simulink model "utpr_model_complex_22"  (R2023b)
settings: Solver=FixedStepAuto  StartTime=0  StopTime=8  FixedStep=0.01  RelTol=1e-2  AbsTol=1e-3  EnableMultiTasking=on
values from neighbouring files (symbols this model uses):
  link1_m = 1.915 * (rand_para(1,1) + 1)    [utpr_model_complex_para.m]
  link2_m = 1.469 * (rand_para(3,1) + 1)    [utpr_model_complex_para.m]
  link3_m = 1.141 * (rand_para(5,1) + 1)    [utpr_model_complex_para.m]
  N = 50    [utpr_lqr.m]    (also in utpr_mpc.m = 100)
undefined symbols (not defined in the file or in its folder): X, Y, Z
libraries: sm_lib x28, nesl_utility x24, simulink x1
settings Model: Creator=李东昊  LastModifiedBy=12720
settings SolverCC: AutoScaleAbsTol=off  AlgebraicLoopSolver=TrustRegion  MaxZcPerStep=1
settings DataIOCC: LimitDataPoints=on  MaxDataPoints=10000
settings OptimizationCC: ReuseModelBlockBuffer=off  LifeSpan=inf
settings DebuggingCC: UnconnectedInputMsg=warning  UnconnectedOutputMsg=warning  UnconnectedLineMsg=warning  AllowSymbolicDim=off  SFUnexpectedBacktrackingDiag=warning  SFNoUnconditionalDefaultTransitionDiag=warning  SFExecutionAtInitializationDiag=none  ArithmeticOperatorsInVariantConditions=warning
settings ModelReferenceCC: EnableRefExpFcnMdlSchedulingChecks=on
settings SFSimCC: SimUseLocalCustomCode=off  CustomCodeUndefinedFunction=UseInterfaceOnly
settings RTWCC: RTWUseLocalCustomCode=off  DLArmComputeVersion=19.05
settings CodeAppCC: StateflowObjectComments=on
settings GRTTargetCC: TargetLangStandard=C89/C90 (ANSI)
settings ConfigComp: CovMetricSettings=dw  CovSaveCumulativeToWorkspaceVar=on  CovSaveSingleToWorkspaceVar=on  CovExternalEMLEnable=off  CovSFcnEnable=off
settings SimscapeCC: SimscapeLogType=all  SimscapeLogSimulationStatistics=on  SimscapeLogDataHistory=10000
settings ExplorerConfigSet: InternalSimMechanicsExplorerSettings="<ExplorerConfiguration><canonicalview>aerospace</canonicalview><AnimationSetting><BasePlaybackSpeed>1.0</BasePlaybackSpeed><PlaybackSpeedFactor>1.0</PlaybackSpeedFactor></AnimationSetting><TilePanel><TileInfo><Tiles Columns=\"1\" Count=\"1\" Rows=\"1\"><Column Weight=\"1\"/><Row Weight=\"1\"/><Tile Height=\"1\" Width=\"1\" X=\"0\" Y=\"0\"/></Tiles></TileInfo><SceneInfo><SceneViewer><BGColor><R>0.60000002384185791</R><G>0.60000002384185791</G><B>0.60000002384185791</B></BGColor><Camera><DoPerspective>off</DoPerspective><Position><X>-0.471212034882517727</X><Y>0.213512906624389098</Y><Z>1.00000005247557366</Z></Position><Center><X>-0.471212034882517727</X><Y>0.213512906624389098</Y><Z>5.24755735531456935e-08</Z></Center><Up><X>0</X><Y>1</Y><Z>0</Z></Up><ViewLimDist>1</ViewLimDist><YLim>1.41406501065933288</YLim><XLim>1.62924881662923138</XLim></Camera></SceneViewer></SceneInfo></TilePanel><MechEditorPanel><Cameras/><GfxPanelCameraMap/><VideoCreator><PlaybackSpeedRatio>1.0</PlaybackSpeedRatio><FrameRate>30</FrameRate><VideoFormat>MPEG-4</VideoFormat><FrameSize>[800 600]</FrameSize></VideoCreator></MechEditorPanel></ExplorerConfiguration>"

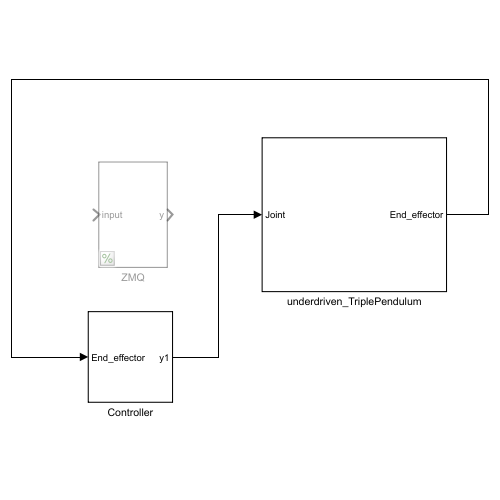
[thumbnail: Simulink's stored preview of the top-level diagram]
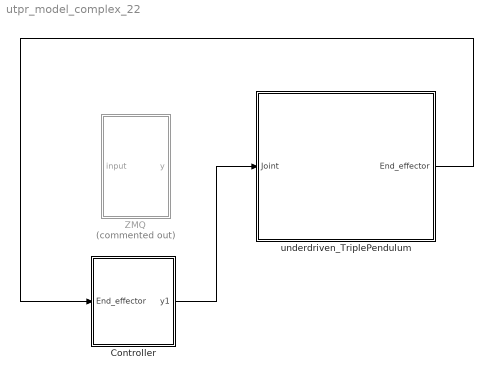
== system utpr_model_complex_22 ==
  Controller : Subsystem
  ZMQ : Subsystem  Commented=on
  underdriven_TriplePendulum : Subsystem
  wires:
  underdriven_TriplePendulum/1(End_effector) -> Controller/1(End_effector)
  Controller/1(y1) -> underdriven_TriplePendulum/1(Joint)

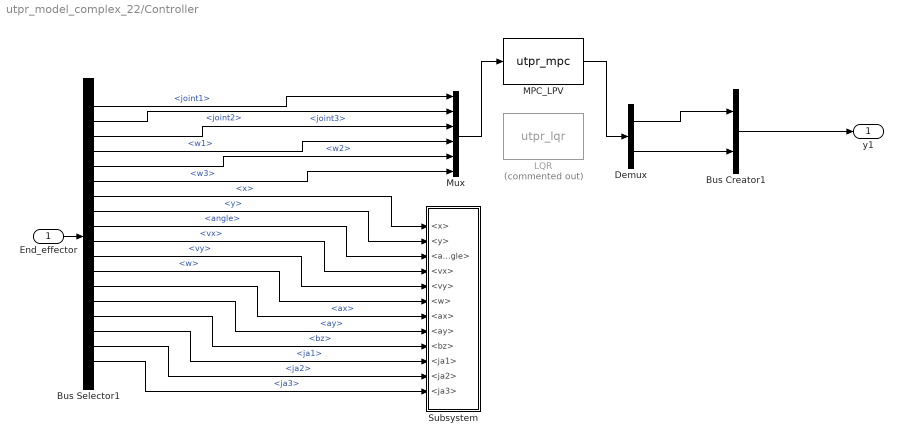
== system utpr_model_complex_22/Controller ==
  End_effector : Inport
  Bus Creator1 : BusCreator  Inputs=2
  Bus Selector1 : BusSelector  OutputSignals=joint1,joint2,joint3,w1,w2,w3,signal1.x,signal1.y,signal1.angle,signal1.vx,signal1.vy,signal1.w,signal1.ax,signal1.ay,signal1.bz,ja1,ja2,ja3
  Demux : Demux  Outputs=2
  LQR : MATLABFcn  Commented=on  MATLABFcn=utpr_lqr  OutputDimensions=2
  MPC_LPV : MATLABFcn  MATLABFcn=utpr_mpc  OutputDimensions=2
  Mux : Mux  Inputs=6
  Subsystem : Subsystem
  y1 : Outport
  wires:
  Bus Creator1/1 -> y1/1
  Bus Selector1/5 -> Mux/5  "<w2>"
  Demux/2 -> Bus Creator1/2
  Bus Selector1/13 -> Subsystem/7(<ax>)  "<ax>"
  Bus Selector1/8 -> Subsystem/2(<y>)  "<y>"
  Bus Selector1/15 -> Subsystem/9(<bz>)  "<bz>"
  Bus Selector1/4 -> Mux/4  "<w1>"
  Bus Selector1/3 -> Mux/3  "<joint3>"
  Bus Selector1/9 -> Subsystem/3(<angle>)  "<angle>"
  Bus Selector1/6 -> Mux/6  "<w3>"
  End_effector/1 -> Bus Selector1/1
  Bus Selector1/10 -> Subsystem/4(<vx>)  "<vx>"
  Bus Selector1/17 -> Subsystem/11(<ja2>)  "<ja2>"
  Bus Selector1/14 -> Subsystem/8(<ay>)  "<ay>"
  Bus Selector1/18 -> Subsystem/12(<ja3>)  "<ja3>"
  Bus Selector1/2 -> Mux/2  "<joint2>"
  Demux/1 -> Bus Creator1/1
  Bus Selector1/16 -> Subsystem/10(<ja1>)  "<ja1>"
  Bus Selector1/11 -> Subsystem/5(<vy>)  "<vy>"
  Bus Selector1/1 -> Mux/1  "<joint1>"
  Bus Selector1/7 -> Subsystem/1(<x>)  "<x>"
  Bus Selector1/12 -> Subsystem/6(<w>)  "<w>"
  Mux/1 -> MPC_LPV/1
  MPC_LPV/1 -> Demux/1

== system utpr_model_complex_22/ZMQ ==
  input : Inport
  Bus Creator2 : BusCreator  Inputs=2
  Bus Selector2 : BusSelector  OutputSignals=joint1,joint2,joint3,w1,w2,w3,signal1.x,signal1.y,signal1.angle,signal1.vx,signal1.vy,signal1.w,signal1.ax,signal1.ay,signal1.bz,ja1,ja2,ja3
  ControlClient : S-Function  FunctionName=controluntriplnsfun  Parameters=hostname,portname,stepsize,inputnum,outputnum  SFunctionDeploymentMode=off  EnableBusSupport=off  mask{hostname=localhost, portname=8099, stepsize=0.01, inputnum=7, outputnum=2}
      mask prompts: hostname "host"; portname "port"; stepsize "step"; inputnum "input num"; outputnum "output num"
      mask DialogControl ParameterGroupVar Prompt: 参数
      mask Display:
      | color('red');
      | image('Simulink_Logo.png');
  y : Outport
  wires:
  Bus Selector2/18 -> ControlClient/18  "<ja3>"
  Bus Selector2/17 -> ControlClient/17  "<ja2>"
  ControlClient/2 -> Bus Creator2/2
  Bus Selector2/12 -> ControlClient/12  "<w>"
  Bus Selector2/6 -> ControlClient/6  "<w3>"
  Bus Selector2/4 -> ControlClient/4  "<w1>"
  Bus Selector2/1 -> ControlClient/1  "<joint1>"
  Bus Selector2/5 -> ControlClient/5  "<w2>"
  Bus Selector2/13 -> ControlClient/13  "<ax>"
  Bus Selector2/14 -> ControlClient/14  "<ay>"
  Bus Selector2/7 -> ControlClient/7  "<x>"
  Bus Selector2/10 -> ControlClient/10  "<vx>"
  Bus Selector2/9 -> ControlClient/9  "<angle>"
  Bus Selector2/15 -> ControlClient/15  "<bz>"
  Bus Selector2/11 -> ControlClient/11  "<vy>"
  Bus Selector2/8 -> ControlClient/8  "<y>"
  Bus Selector2/3 -> ControlClient/3  "<joint3>"
  Bus Selector2/16 -> ControlClient/16  "<ja1>"
  input/1 -> Bus Selector2/1
  Bus Selector2/2 -> ControlClient/2  "<joint2>"
  Bus Creator2/1 -> y/1
  ControlClient/1 -> Bus Creator2/1

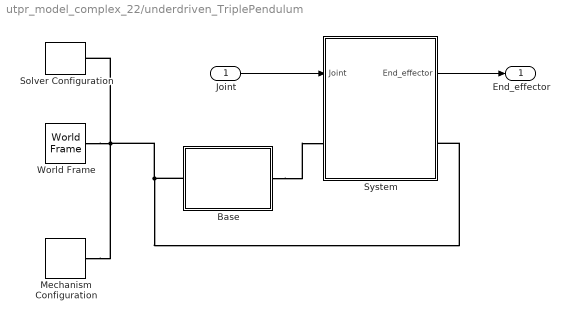
== system utpr_model_complex_22/underdriven_TriplePendulum ==
  Joint : Inport
  Base : Subsystem  mask{R=10, T=0.5, rp=1}
      mask prompts: R "base rasuis（cm）"; T "Base thickness (cm):"; rp "Peg radius（cm）"
      mask DialogControl ParameterGroupVar Prompt: 参数
      mask Display: image('utpr_base.png');
  Mechanism Configuration : sm_lib/Utilities/Mechanism Configuration  UniformGravity=Constant  GravityVector=[0 -9.81 0]  GravityVectorUnits=m/s^2  LinearizationDelta=0.01  JointModeTransitionNonlinearIterations=2
  Solver Configuration : nesl_utility/Solver Configuration  PhysicalDomain=network_engine_domain  SubClassName=solver  LeftPortType=input  RightPortType=generic  Tones=[]  Harmonics=[]  SimulateNoise=off  Profile=off  UseLocalSampling=off  EnableSwitchedLinearOptims=on  FrequencyDomain=off  UseCCode=off  RelTol=0.001  AbsTol=1e-06  MinStep=1e-09  ToWorkspace=off  RevertToSquareIcSolve=off  NumHomotopyIterations=100  PhasorMode=off  PhasorModeNumHarmonics=1  ConsistencySolver=NEWTON_FTOL  IndexReductionMethod=DerivativeReplacement  DoDC=off  ResidualTolerance=1e-09  ConsistencyTolSource=GLOBAL  ConsistencyAbsTol=0.001  ConsistencyRelTol=0.001  ConsistencyTolFactor=0.001  UseLocalSolver=off  LocalSolverChoice=NE_BACKWARD_EULER_ADVANCER  ResolveIndetEquations=on  FunctionEvalNumThread=1  LocalSolverSampleTime=0.001  DoFixedCost=off  MaxNonlinIter=3  MaxModeIter=2  ComputeImpulses=off  ImpulseIterations=2  LinearAlgebra=Sparse  LinearAlgebraNumThread=0  EquationFormulation=NE_TIME_EF  DelaysMemoryBudget=1024  AutomaticFiltering=on  FilteringTimeConstant=0.01  PartitionStorageMethod=AS_NEEDED  PartitionMemoryBudget=1024  PartitionMethod=FAST  MultibodyUseLocalSolver=off  MultibodyLocalSolverChoice=ODE1  MultibodyLocalSolverSampleTime=0.001
  System : Subsystem
  World Frame : sm_lib/Frames and Transforms/World Frame
  End_effector : Outport
  wires:
  System/1(End_effector) -> End_effector/1
  Joint/1 -> System/1(Joint)
  connections:
  World Frame/RConn1 -- System/RConn1 -- Base/LConn1 -- Mechanism Configuration/RConn1 -- Solver Configuration/RConn1
  Base/RConn1 -- System/LConn1

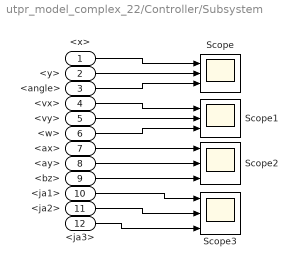
== system utpr_model_complex_22/Controller/Subsystem ==
  <x> : Inport
  <y> : Inport  Port=2
  <angle> : Inport  Port=3
  <vx> : Inport  Port=4
  <vy> : Inport  Port=5
  <w> : Inport  Port=6
  <ax> : Inport  Port=7
  <ay> : Inport  Port=8
  <bz> : Inport  Port=9
  <ja1> : Inport  Port=10
  <ja2> : Inport  Port=11
  <ja3> : Inport  Port=12
  Scope{,1..3} (4 alike) : Scope  NumInputPorts=3
  wires:
  <y>/1 -> Scope/2
  <ja1>/1 -> Scope3/1
  <bz>/1 -> Scope2/3
  <ax>/1 -> Scope2/1
  <vy>/1 -> Scope1/2
  <x>/1 -> Scope/1
  <angle>/1 -> Scope/3
  <ja2>/1 -> Scope3/2
  <ay>/1 -> Scope2/2
  <w>/1 -> Scope1/3
  <vx>/1 -> Scope1/1
  <ja3>/1 -> Scope3/3

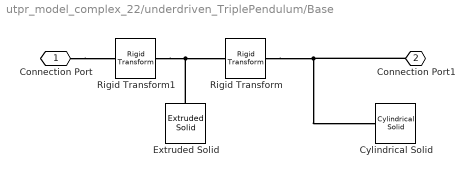
== system utpr_model_complex_22/underdriven_TriplePendulum/Base ==
  Cylindrical Solid : sm_lib/Body Elements/Cylindrical Solid  CylinderRadius=rp  CylinderRadiusUnits=cm  CylinderLength=2*T  CylinderLengthUnits=cm  ExportEntireGeometry=off  InertiaType=CalculateFromGeometry  BasedOnType=Density  Density=1  DensityUnits=kg/m^3  Mass=1  MassUnits=kg  CenterOfMass=[0 0 0]  CenterOfMassUnits=m  MomentsOfInertia=[1 1 1]  MomentsOfInertiaUnits=kg*m^2  ProductsOfInertia=[0 0 0]  ProductsOfInertiaUnits=kg*m^2  GraphicType=FromGeometry  MarkerShape=Sphere  MarkerSize=10  GraphicVisPropType=SimpleVisualProperties  GraphicDiffuseColor=[0.2 0.2 0.2]  GraphicOpacity=1  GraphicSpecularColor=[0.5 0.5 0.5 1.0]  GraphicAmbientColor=[0.15 0.15 0.15 1.0]  GraphicEmissiveColor=[0.0 0.0 0.0 1.0]  GraphicShininess=75  DoExposeReferenceFrame=on  SerializedFrames=<Frames/>
  Extruded Solid : sm_lib/Body Elements/Extruded Solid  ExtrusionType=Regular  PolygonNumSides=6  PolygonOuterRadius=R  PolygonOuterRadiusUnits=cm  ExportEntireGeometry=off  ExtrusionCrossSection=[1 1; -1 1; -1 -1; 1 -1]  ExtrusionCrossSectionUnits=m  ExportConvexHullGeometry=off  ExtrusionLength=T  ExtrusionLengthUnits=cm  InertiaType=CalculateFromGeometry  BasedOnType=Density  Density=1  DensityUnits=kg/m^3  Mass=1  MassUnits=kg  CenterOfMass=[0 0 0]  CenterOfMassUnits=m  MomentsOfInertia=[1 1 1]  MomentsOfInertiaUnits=kg*m^2  ProductsOfInertia=[0 0 0]  ProductsOfInertiaUnits=kg*m^2  GraphicType=FromGeometry  MarkerShape=Sphere  MarkerSize=10  GraphicVisPropType=SimpleVisualProperties  GraphicDiffuseColor=[0.2 0.2 0.2]  GraphicOpacity=1  GraphicSpecularColor=[0.5 0.5 0.5 1.0]  GraphicAmbientColor=[0.15 0.15 0.15 1.0]  GraphicEmissiveColor=[0.0 0.0 0.0 1.0]  GraphicShininess=75  DoExposeReferenceFrame=on  SerializedFrames=<Frames/>
  Rigid Transform : sm_lib/Frames and Transforms/Rigid Transform  RotationMethod=None  FollAlignAxisA=+X  BaseAlignAxisA=+Y  FollAlignAxisB=+Y  BaseAlignAxisB=+Z  RotationStandardAxis=+Z  RotationAngle=0  RotationAngleUnits=deg  RotationArbitraryAxis=[0 0 1]  RotationSequenceAxes=FollowerAxes  RotationSequence=XYX  RotationSequenceAngles=[0 0 0]  RotationSequenceAnglesUnits=deg  RotationMatrix=[1 0 0;0 1 0;0 0 1]  Quaternion=[1 0 0 0]  TranslationMethod=StandardAxis  TranslationCartesianOffset=[0 0 0]  TranslationCartesianOffsetUnits=m  TranslationStandardAxis=+Z  TranslationStandardOffset=3*T/2  TranslationStandardOffsetUnits=cm  TranslationROffset=0  TranslationROffsetUnits=m  TranslationThetaOffset=0  TranslationThetaOffsetUnits=deg  TranslationZOffset=0  TranslationZOffsetUnits=m
  Rigid Transform1 : sm_lib/Frames and Transforms/Rigid Transform  RotationMethod=None  FollAlignAxisA=+Z  BaseAlignAxisA=-Y  FollAlignAxisB=+Y  BaseAlignAxisB=+X  RotationStandardAxis=+Z  RotationAngle=0  RotationAngleUnits=deg  RotationArbitraryAxis=[0 0 1]  RotationSequenceAxes=FollowerAxes  RotationSequence=XYX  RotationSequenceAngles=[0 0 0]  RotationSequenceAnglesUnits=deg  RotationMatrix=[1 0 0;0 1 0;0 0 1]  Quaternion=[1 0 0 0]  TranslationMethod=StandardAxis  TranslationCartesianOffset=[0 0 0]  TranslationCartesianOffsetUnits=m  TranslationStandardAxis=+Z  TranslationStandardOffset=-T  TranslationStandardOffsetUnits=cm  TranslationROffset=0  TranslationROffsetUnits=m  TranslationThetaOffset=0  TranslationThetaOffsetUnits=deg  TranslationZOffset=0  TranslationZOffsetUnits=m
  Connection Port : PMIOPort  Side=Left
  Connection Port1 : PMIOPort  Port=2  Side=Right
  connections:
  Extruded Solid/RConn1 -- Rigid Transform1/RConn1 -- Rigid Transform/LConn1
  Rigid Transform/RConn1 -- Cylindrical Solid/RConn1 -- Connection Port1/RConn1
  Connection Port/RConn1 -- Rigid Transform1/LConn1

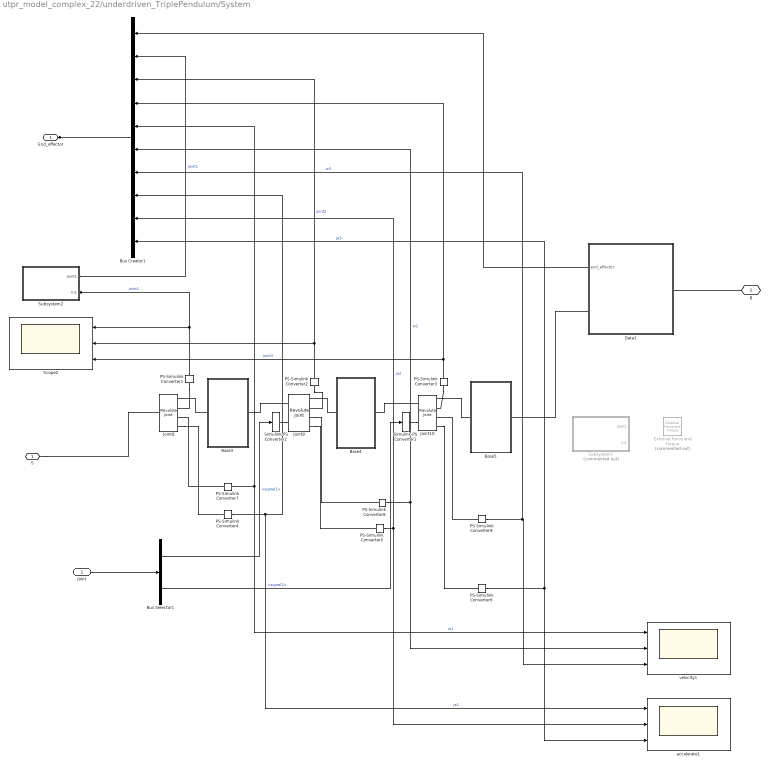
== system utpr_model_complex_22/underdriven_TriplePendulum/System ==
  Joint : Inport
  Base3 : Subsystem  mask{R=6, T=0.5, rp=1, link1_rgb=[0.8 0.2 0.0]}
      mask prompts: R "base rasuis（cm）"; T "Base thickness (cm):"; rp "Peg radius（cm）"; link1_rgb "link color"
      mask DialogControl ParameterGroupVar Prompt: 参数
      mask Display: image('utpr_link1.png');
  Base4 : Subsystem  mask{R=6, T=0.5, rp=1, link1_rgb=[1.0 0.8 0.0]}
      mask prompts: R "base rasuis（cm）"; T "Base thickness (cm):"; rp "Peg radius（cm）"; link1_rgb "link color"
      mask DialogControl ParameterGroupVar Prompt: 参数
      mask Display: image('utpr_link1.png');
  Base5 : Subsystem  mask{R=6, T=0.5, rp=1, link1_rgb=[0.0 0.6 0.2 ]}
      mask prompts: R "base rasuis（cm）"; T "Base thickness (cm):"; rp "Peg radius（cm）"; link1_rgb "link color"
      mask DialogControl ParameterGroupVar Prompt: 参数
      mask Display: image('utpr_link1.png');
  Bus Creator1 : BusCreator  Inputs=10
  Bus Selector1 : BusSelector  OutputSignals=signal1,signal2
  Data1 : Subsystem
  External Force and Torque : sm_lib/Forces and Torques/External Force and Torque  Commented=on  EnableForceX=on  EnableForceY=off  EnableForceZ=off  EnableForce=off  ForceResolutionFrame=World  EnableTorqueX=off  EnableTorqueY=off  EnableTorqueZ=off  EnableTorque=off  TorqueResolutionFrame=AttachedFrame
  Joint10 : sm_lib/Joints/Revolute Joint  JointMode=Normal  CompositeWrenchDir=BaseOnFollower  CompositeWrenchFrame=BaseFrame  SenseConstraintForce=off  SenseConstraintTorque=off  SenseTotalForce=off  SenseTotalTorque=off  PositionTargetSpecify=on  PositionTargetPriority=High  PositionTargetValue=0.6  PositionTargetValueUnits=deg  VelocityTargetSpecify=off  VelocityTargetPriority=High  VelocityTargetValue=0  VelocityTargetValueUnits=rad/s  EquilibriumPosition=0  EquilibriumPositionUnits=deg  SpringStiffness=0  SpringStiffnessUnits=N*m/deg  DampingCoefficient=0  DampingCoefficientUnits=N*m/(deg/s)  LowerLimitSpecify=off  LowerLimitBound=-90  LowerLimitBoundUnits=deg  LowerLimitStiffness=1e4  LowerLimitStiffnessUnits=N*m/deg  LowerLimitDamping=10  LowerLimitDampingUnits=N*m/(deg/s)  LowerLimitTransitionRegionWidth=0.1  LowerLimitTransitionRegionWidthUnits=deg  UpperLimitSpecify=off  UpperLimitBound=90  UpperLimitBoundUnits=deg  UpperLimitStiffness=1e4  UpperLimitStiffnessUnits=N*m/deg  UpperLimitDamping=10  UpperLimitDampingUnits=N*m/(deg/s)  UpperLimitTransitionRegionWidth=0.1  UpperLimitTransitionRegionWidthUnits=deg  TorqueActuationMode=InputTorque  MotionActuationMode=ComputedMotion  SensePosition=on  SenseVelocity=on  SenseAcceleration=on  SenseTorqueForce=off  SenseLowerLimitTorqueForce=off  SenseUpperLimitTorqueForce=off
  Joint8 : sm_lib/Joints/Revolute Joint  JointMode=Normal  CompositeWrenchDir=BaseOnFollower  CompositeWrenchFrame=BaseFrame  SenseConstraintForce=off  SenseConstraintTorque=off  SenseTotalForce=off  SenseTotalTorque=off  PositionTargetSpecify=on  PositionTargetPriority=High  PositionTargetValue=0.6  PositionTargetValueUnits=deg  VelocityTargetSpecify=off  VelocityTargetPriority=Low  VelocityTargetValue=0  VelocityTargetValueUnits=rad/s  EquilibriumPosition=0  EquilibriumPositionUnits=deg  SpringStiffness=0  SpringStiffnessUnits=N*m/deg  DampingCoefficient=0  DampingCoefficientUnits=N*m/(deg/s)  LowerLimitSpecify=off  LowerLimitBound=-90  LowerLimitBoundUnits=deg  LowerLimitStiffness=1e4  LowerLimitStiffnessUnits=N*m/deg  LowerLimitDamping=10  LowerLimitDampingUnits=N*m/(deg/s)  LowerLimitTransitionRegionWidth=0.1  LowerLimitTransitionRegionWidthUnits=deg  UpperLimitSpecify=off  UpperLimitBound=90  UpperLimitBoundUnits=deg  UpperLimitStiffness=1e4  UpperLimitStiffnessUnits=N*m/deg  UpperLimitDamping=10  UpperLimitDampingUnits=N*m/(deg/s)  UpperLimitTransitionRegionWidth=0.1  UpperLimitTransitionRegionWidthUnits=deg  TorqueActuationMode=NoTorque  MotionActuationMode=ComputedMotion  SensePosition=on  SenseVelocity=on  SenseAcceleration=on  SenseTorqueForce=off  SenseLowerLimitTorqueForce=off  SenseUpperLimitTorqueForce=off
  Joint9 : sm_lib/Joints/Revolute Joint  JointMode=Normal  CompositeWrenchDir=BaseOnFollower  CompositeWrenchFrame=BaseFrame  SenseConstraintForce=off  SenseConstraintTorque=off  SenseTotalForce=off  SenseTotalTorque=off  PositionTargetSpecify=on  PositionTargetPriority=High  PositionTargetValue=0.6  PositionTargetValueUnits=deg  VelocityTargetSpecify=off  VelocityTargetPriority=High  VelocityTargetValue=0  VelocityTargetValueUnits=rad/s  EquilibriumPosition=0  EquilibriumPositionUnits=deg  SpringStiffness=0  SpringStiffnessUnits=N*m/deg  DampingCoefficient=0  DampingCoefficientUnits=N*m/(deg/s)  LowerLimitSpecify=off  LowerLimitBound=-90  LowerLimitBoundUnits=rad  LowerLimitStiffness=0  LowerLimitStiffnessUnits=N*m/deg  LowerLimitDamping=0  LowerLimitDampingUnits=N*m/(deg/s)  LowerLimitTransitionRegionWidth=0.0  LowerLimitTransitionRegionWidthUnits=deg  UpperLimitSpecify=off  UpperLimitBound=90  UpperLimitBoundUnits=deg  UpperLimitStiffness=1e4  UpperLimitStiffnessUnits=N*m/deg  UpperLimitDamping=10  UpperLimitDampingUnits=N*m/(deg/s)  UpperLimitTransitionRegionWidth=0.1  UpperLimitTransitionRegionWidthUnits=deg  TorqueActuationMode=InputTorque  MotionActuationMode=ComputedMotion  SensePosition=on  SenseVelocity=on  SenseAcceleration=on  SenseTorqueForce=off  SenseLowerLimitTorqueForce=off  SenseUpperLimitTorqueForce=off
  PS-Simulink Converter{1..9} (9 alike) : nesl_utility/PS-Simulink Converter  PhysicalDomain=network_engine_domain  SubClassName=ps_output  LeftPortType=input  RightPortType=output  PseudoPeriodic=off  Frequencies=[]  VectorFormat=inherit  Unit=inherit  AffineConversion=off
  Scope2 : Scope  NumInputPorts=3
  Simulink-PS Converter1 : nesl_utility/Simulink-PS Converter  PhysicalDomain=network_engine_domain  SubClassName=ps_input  LeftPortType=input  RightPortType=output  PseudoPeriodic=off  Frequencies=[]  NoiseDistribution=none  NoiseParameters=[]  Unit=1  AffineConversion=off  FilteringAndDerivatives=provide  SimscapeFilterOrder=2  InputFilterTimeConstant=0.001  UdotUserProvided=0
  Simulink-PS Converter2 : nesl_utility/Simulink-PS Converter  PhysicalDomain=network_engine_domain  SubClassName=ps_input  LeftPortType=input  RightPortType=output  PseudoPeriodic=off  Frequencies=[]  NoiseDistribution=none  NoiseParameters=[]  Unit=1  AffineConversion=off  FilteringAndDerivatives=provide  SimscapeFilterOrder=2  InputFilterTimeConstant=0.001  UdotUserProvided=0
  Subsystem1 : Subsystem  Commented=on
      settings: PortSchema="{\"entries\":[{\"content\":{\"sides\":[{\"content\":{},\"type\":\"ConnectorPlacement.EquallySpacedRectSide\",\"uuid\":\"6104612b-0199-40d9-be5b-c88f2ec8b275\"},{\"content\":{\"connectorIds\":[\"Out1\",\"In1\"],\"side\":\"RIGHT\"},\"type\":\"ConnectorPlacement.EquallySpacedRectSide\",\"uuid\":\"49652b33-c69d-46aa-bdcb-b7d535b54a7f\"},{\"content\":{\"side\":\"TOP\"},\"type\":\"ConnectorPlacement.EquallySpacedRectSide\",\"uuid\":\"a81b527b-df77-41c9-ae60-18d5269f8c84\"}]},\"type\":\"ConnectorPlacement.EquallySpacedConnector\",\"uuid\":\"40a92e28-c47c-4b9d-90cf-16ea482bd807\"}],\"packageUris\":[\"http://schema.mathworks.com/mf0/Connector/R2020b\"],\"version\":\"1.0\"}"
  Subsystem2 : Subsystem
      settings: PortSchema="{\"entries\":[{\"content\":{\"sides\":[{\"content\":{},\"type\":\"ConnectorPlacement.EquallySpacedRectSide\",\"uuid\":\"6104612b-0199-40d9-be5b-c88f2ec8b275\"},{\"content\":{\"connectorIds\":[\"Out1\",\"In1\"],\"side\":\"RIGHT\"},\"type\":\"ConnectorPlacement.EquallySpacedRectSide\",\"uuid\":\"49652b33-c69d-46aa-bdcb-b7d535b54a7f\"},{\"content\":{\"side\":\"TOP\"},\"type\":\"ConnectorPlacement.EquallySpacedRectSide\",\"uuid\":\"a81b527b-df77-41c9-ae60-18d5269f8c84\"}]},\"type\":\"ConnectorPlacement.EquallySpacedConnector\",\"uuid\":\"40a92e28-c47c-4b9d-90cf-16ea482bd807\"}],\"packageUris\":[\"http://schema.mathworks.com/mf0/Connector/R2020b\"],\"version\":\"1.0\"}"
  accelerate1 : Scope  NumInputPorts=3
  velocity1 : Scope  NumInputPorts=3
  S : PMIOPort  Side=Left
  B : PMIOPort  Port=2  Side=Right
  End_effector : Outport
  wires:
  Data1/1(end_effector) -> Bus Creator1/1
  PS-Simulink Converter1/1 -> Subsystem2/1(In1), Scope2/1  "joint1"
  PS-Simulink Converter5/1 -> accelerate1/2, Bus Creator1/9  "ja2"
  PS-Simulink Converter2/1 -> Bus Creator1/3, Scope2/2  "joint2"
  PS-Simulink Converter8/1 -> Bus Creator1/6, velocity1/2  "w2"
  PS-Simulink Converter7/1 -> Bus Creator1/5, velocity1/1  "w1"
  PS-Simulink Converter4/1 -> accelerate1/1, Bus Creator1/8  "ja1"
  Bus Selector1/1 -> Simulink-PS Converter2/1  "<signal1>"
  Bus Selector1/2 -> Simulink-PS Converter1/1  "<signal2>"
  PS-Simulink Converter6/1 -> Bus Creator1/10, accelerate1/3  "ja3"
  PS-Simulink Converter9/1 -> Bus Creator1/7, velocity1/3  "w3"
  Bus Creator1/1 -> End_effector/1
  Joint/1 -> Bus Selector1/1
  PS-Simulink Converter3/1 -> Bus Creator1/4, Scope2/3  "joint3"
  Subsystem2/1(joint1) -> Bus Creator1/2  "joint1"
  connections:
  Joint10/RConn1 -- Base5/LConn1
  Data1/RConn1 -- Base5/RConn1
  Joint9/RConn3 -- PS-Simulink Converter8/LConn1
  Simulink-PS Converter1/RConn1 -- Joint10/LConn2
  B/RConn1 -- Data1/LConn1
  Joint8/RConn4 -- PS-Simulink Converter4/LConn1
  Joint10/RConn4 -- PS-Simulink Converter6/LConn1
  Joint10/LConn1 -- Base4/RConn1
  PS-Simulink Converter9/LConn1 -- Joint10/RConn3
  PS-Simulink Converter2/LConn1 -- Joint9/RConn2
  Joint9/RConn4 -- PS-Simulink Converter5/LConn1
  PS-Simulink Converter1/LConn1 -- Joint8/RConn2
  Base3/LConn1 -- Joint8/RConn1
  Base3/RConn1 -- Joint9/LConn1
  PS-Simulink Converter7/LConn1 -- Joint8/RConn3
  PS-Simulink Converter3/LConn1 -- Joint10/RConn2
  S/RConn1 -- Joint8/LConn1
  Base4/LConn1 -- Joint9/RConn1
  Simulink-PS Converter2/RConn1 -- Joint9/LConn2

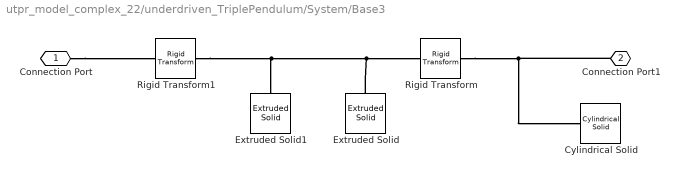
== system utpr_model_complex_22/underdriven_TriplePendulum/System/Base3 ==
  Cylindrical Solid : sm_lib/Body Elements/Cylindrical Solid  CylinderRadius=rp  CylinderRadiusUnits=cm  CylinderLength=2*T  CylinderLengthUnits=cm  ExportEntireGeometry=off  InertiaType=PointMass  BasedOnType=Density  Density=1  DensityUnits=kg/m^3  Mass=1e-20  MassUnits=kg  CenterOfMass=[0 0 0]  CenterOfMassUnits=m  MomentsOfInertia=[1 1 1]  MomentsOfInertiaUnits=kg*m^2  ProductsOfInertia=[0 0 0]  ProductsOfInertiaUnits=kg*m^2  GraphicType=FromGeometry  MarkerShape=Sphere  MarkerSize=10  GraphicVisPropType=SimpleVisualProperties  GraphicDiffuseColor=link1_rgb  GraphicOpacity=1  GraphicSpecularColor=[0.5 0.5 0.5 1.0]  GraphicAmbientColor=[0.15 0.15 0.15 1.0]  GraphicEmissiveColor=[0.0 0.0 0.0 1.0]  GraphicShininess=75  DoExposeReferenceFrame=on  SerializedFrames=<Frames/>
  Extruded Solid : sm_lib/Body Elements/Extruded Solid  ExtrusionType=General  PolygonNumSides=6  PolygonOuterRadius=R  PolygonOuterRadiusUnits=cm  ExportEntireGeometry=off  ExtrusionCrossSection=link1_section  ExtrusionCrossSectionUnits=m  ExportConvexHullGeometry=off  ExtrusionLength=T  ExtrusionLengthUnits=cm  InertiaType=Custom  BasedOnType=Density  Density=1  DensityUnits=kg/m^3  Mass=link1_m  MassUnits=kg  CenterOfMass=link1_CM  CenterOfMassUnits=m  MomentsOfInertia=link1_MI  MomentsOfInertiaUnits=kg*m^2  ProductsOfInertia=[0 0 0]  ProductsOfInertiaUnits=kg*m^2  GraphicType=FromGeometry  MarkerShape=Sphere  MarkerSize=10  GraphicVisPropType=SimpleVisualProperties  GraphicDiffuseColor=link1_rgb  GraphicOpacity=1  GraphicSpecularColor=[0.5 0.5 0.5 1.0]  GraphicAmbientColor=[0.15 0.15 0.15 1.0]  GraphicEmissiveColor=[0.0 0.0 0.0 1.0]  GraphicShininess=75  DoExposeReferenceFrame=on  SerializedFrames=<Frames/>
  Extruded Solid1 : sm_lib/Body Elements/Extruded Solid  ExtrusionType=General  PolygonNumSides=6  PolygonOuterRadius=R  PolygonOuterRadiusUnits=cm  ExportEntireGeometry=off  ExtrusionCrossSection=left_end_x_section  ExtrusionCrossSectionUnits=m  ExportConvexHullGeometry=off  ExtrusionLength=T  ExtrusionLengthUnits=cm  InertiaType=PointMass  BasedOnType=Density  Density=1  DensityUnits=kg/m^3  Mass=1e-20  MassUnits=kg  CenterOfMass=[0 0 0]  CenterOfMassUnits=m  MomentsOfInertia=[1 1 1]  MomentsOfInertiaUnits=kg*m^2  ProductsOfInertia=[0 0 0]  ProductsOfInertiaUnits=kg*m^2  GraphicType=FromGeometry  MarkerShape=Sphere  MarkerSize=10  GraphicVisPropType=SimpleVisualProperties  GraphicDiffuseColor=link1_rgb  GraphicOpacity=1  GraphicSpecularColor=[0.5 0.5 0.5 1.0]  GraphicAmbientColor=[0.15 0.15 0.15 1.0]  GraphicEmissiveColor=[0.0 0.0 0.0 1.0]  GraphicShininess=75  DoExposeReferenceFrame=off  SerializedFrames=<Frames><Frame><Id>Frame1</Id><Value><Name>F1</Name><Origin><Source>ReferenceFrame</Source><FeatureName></FeatureName></Origin><PrimaryAxis><DefinedDirection>+Z</DefinedDirection><Source>ReferenceFrame</Source><SourceDirection>+Z</SourceDirection><FeatureName></FeatureName></PrimaryAxis><SecondaryAxis><DefinedDirection>+X</DefinedDirection><Source>ReferenceFrame</Source><SourceDirection>-X</SourceDirection><FeatureName></FeatureName></SecondaryAxis></Value></Frame></Frames>
  Rigid Transform : sm_lib/Frames and Transforms/Rigid Transform  RotationMethod=None  FollAlignAxisA=+X  BaseAlignAxisA=+Y  FollAlignAxisB=+Y  BaseAlignAxisB=+Z  RotationStandardAxis=+Z  RotationAngle=0  RotationAngleUnits=deg  RotationArbitraryAxis=[0 0 1]  RotationSequenceAxes=FollowerAxes  RotationSequence=XYX  RotationSequenceAngles=[0 0 0]  RotationSequenceAnglesUnits=deg  RotationMatrix=[1 0 0;0 1 0;0 0 1]  Quaternion=[1 0 0 0]  TranslationMethod=StandardAxis  TranslationCartesianOffset=[0 0 0]  TranslationCartesianOffsetUnits=m  TranslationStandardAxis=+X  TranslationStandardOffset=L1  TranslationStandardOffsetUnits=m  TranslationROffset=0  TranslationROffsetUnits=m  TranslationThetaOffset=0  TranslationThetaOffsetUnits=deg  TranslationZOffset=0  TranslationZOffsetUnits=m
  Rigid Transform1 : sm_lib/Frames and Transforms/Rigid Transform  RotationMethod=StandardAxis  FollAlignAxisA=+X  BaseAlignAxisA=+Y  FollAlignAxisB=+Y  BaseAlignAxisB=+Z  RotationStandardAxis=+Z  RotationAngle=90  RotationAngleUnits=deg  RotationArbitraryAxis=[0 0 1]  RotationSequenceAxes=FollowerAxes  RotationSequence=XYX  RotationSequenceAngles=[0 0 0]  RotationSequenceAnglesUnits=deg  RotationMatrix=[1 0 0;0 1 0;0 0 1]  Quaternion=[1 0 0 0]  TranslationMethod=StandardAxis  TranslationCartesianOffset=[0 0 0]  TranslationCartesianOffsetUnits=m  TranslationStandardAxis=+Y  TranslationStandardOffset=0  TranslationStandardOffsetUnits=m  TranslationROffset=0  TranslationROffsetUnits=m  TranslationThetaOffset=0  TranslationThetaOffsetUnits=deg  TranslationZOffset=0  TranslationZOffsetUnits=m
  Connection Port : PMIOPort  Side=Left
  Connection Port1 : PMIOPort  Port=2  Side=Right
  connections:
  Connection Port1/RConn1 -- Rigid Transform/RConn1 -- Cylindrical Solid/RConn1
  Rigid Transform1/RConn1 -- Extruded Solid1/LConn1 -- Extruded Solid/RConn1 -- Rigid Transform/LConn1
  Connection Port/RConn1 -- Rigid Transform1/LConn1

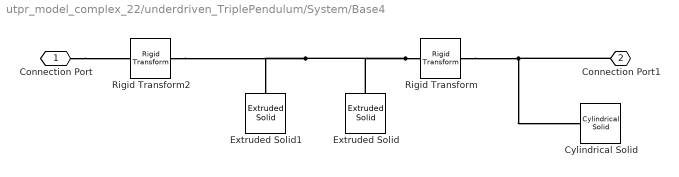
== system utpr_model_complex_22/underdriven_TriplePendulum/System/Base4 ==
  Cylindrical Solid : sm_lib/Body Elements/Cylindrical Solid  CylinderRadius=rp  CylinderRadiusUnits=cm  CylinderLength=2*T  CylinderLengthUnits=cm  ExportEntireGeometry=off  InertiaType=PointMass  BasedOnType=Density  Density=1  DensityUnits=kg/m^3  Mass=1e-20  MassUnits=g  CenterOfMass=[0 0 0]  CenterOfMassUnits=m  MomentsOfInertia=[1 1 1]  MomentsOfInertiaUnits=kg*m^2  ProductsOfInertia=[0 0 0]  ProductsOfInertiaUnits=kg*m^2  GraphicType=FromGeometry  MarkerShape=Sphere  MarkerSize=10  GraphicVisPropType=SimpleVisualProperties  GraphicDiffuseColor=link1_rgb  GraphicOpacity=1  GraphicSpecularColor=[0.5 0.5 0.5 1.0]  GraphicAmbientColor=[0.15 0.15 0.15 1.0]  GraphicEmissiveColor=[0.0 0.0 0.0 1.0]  GraphicShininess=75  DoExposeReferenceFrame=on  SerializedFrames=<Frames/>
  Extruded Solid : sm_lib/Body Elements/Extruded Solid  ExtrusionType=General  PolygonNumSides=6  PolygonOuterRadius=R  PolygonOuterRadiusUnits=cm  ExportEntireGeometry=off  ExtrusionCrossSection=link2_section  ExtrusionCrossSectionUnits=m  ExportConvexHullGeometry=off  ExtrusionLength=T  ExtrusionLengthUnits=cm  InertiaType=Custom  BasedOnType=Density  Density=1  DensityUnits=kg/m^3  Mass=link2_m  MassUnits=kg  CenterOfMass=link2_CM  CenterOfMassUnits=m  MomentsOfInertia=link2_MI  MomentsOfInertiaUnits=kg*m^2  ProductsOfInertia=[0 0 0]  ProductsOfInertiaUnits=kg*m^2  GraphicType=FromGeometry  MarkerShape=Sphere  MarkerSize=10  GraphicVisPropType=SimpleVisualProperties  GraphicDiffuseColor=link1_rgb  GraphicOpacity=1  GraphicSpecularColor=[0.5 0.5 0.5 1.0]  GraphicAmbientColor=[0.15 0.15 0.15 1.0]  GraphicEmissiveColor=[0.0 0.0 0.0 1.0]  GraphicShininess=75  DoExposeReferenceFrame=on  SerializedFrames=<Frames/>
  Extruded Solid1 : sm_lib/Body Elements/Extruded Solid  ExtrusionType=General  PolygonNumSides=6  PolygonOuterRadius=R  PolygonOuterRadiusUnits=cm  ExportEntireGeometry=off  ExtrusionCrossSection=left_end_x_section  ExtrusionCrossSectionUnits=m  ExportConvexHullGeometry=off  ExtrusionLength=T  ExtrusionLengthUnits=cm  InertiaType=PointMass  BasedOnType=Density  Density=1  DensityUnits=kg/m^3  Mass=1e-20  MassUnits=g  CenterOfMass=[0 0 0]  CenterOfMassUnits=m  MomentsOfInertia=[1 1 1]  MomentsOfInertiaUnits=kg*m^2  ProductsOfInertia=[0 0 0]  ProductsOfInertiaUnits=kg*m^2  GraphicType=FromGeometry  MarkerShape=Sphere  MarkerSize=10  GraphicVisPropType=SimpleVisualProperties  GraphicDiffuseColor=link1_rgb  GraphicOpacity=1  GraphicSpecularColor=[0.5 0.5 0.5 1.0]  GraphicAmbientColor=[0.15 0.15 0.15 1.0]  GraphicEmissiveColor=[0.0 0.0 0.0 1.0]  GraphicShininess=75  DoExposeReferenceFrame=off  SerializedFrames=<Frames><Frame><Id>Frame1</Id><Value><Name>F1</Name><Origin><Source>ReferenceFrame</Source><FeatureName></FeatureName></Origin><PrimaryAxis><DefinedDirection>+Z</DefinedDirection><Source>ReferenceFrame</Source><SourceDirection>+Z</SourceDirection><FeatureName></FeatureName></PrimaryAxis><SecondaryAxis><DefinedDirection>+X</DefinedDirection><Source>ReferenceFrame</Source><SourceDirection>-X</SourceDirection><FeatureName></FeatureName></SecondaryAxis></Value></Frame></Frames>
  Rigid Transform : sm_lib/Frames and Transforms/Rigid Transform  RotationMethod=None  FollAlignAxisA=+X  BaseAlignAxisA=+Y  FollAlignAxisB=+Y  BaseAlignAxisB=+Z  RotationStandardAxis=+Z  RotationAngle=0  RotationAngleUnits=deg  RotationArbitraryAxis=[0 0 1]  RotationSequenceAxes=FollowerAxes  RotationSequence=XYX  RotationSequenceAngles=[0 0 0]  RotationSequenceAnglesUnits=deg  RotationMatrix=[1 0 0;0 1 0;0 0 1]  Quaternion=[1 0 0 0]  TranslationMethod=StandardAxis  TranslationCartesianOffset=[0 0 0]  TranslationCartesianOffsetUnits=m  TranslationStandardAxis=+X  TranslationStandardOffset=L2  TranslationStandardOffsetUnits=m  TranslationROffset=0  TranslationROffsetUnits=m  TranslationThetaOffset=0  TranslationThetaOffsetUnits=deg  TranslationZOffset=0  TranslationZOffsetUnits=m
  Rigid Transform2 : sm_lib/Frames and Transforms/Rigid Transform  RotationMethod=None  FollAlignAxisA=+X  BaseAlignAxisA=+X  FollAlignAxisB=-Y  BaseAlignAxisB=+Y  RotationStandardAxis=+Z  RotationAngle=90  RotationAngleUnits=deg  RotationArbitraryAxis=[0 0 1]  RotationSequenceAxes=FollowerAxes  RotationSequence=XYX  RotationSequenceAngles=[0 0 0]  RotationSequenceAnglesUnits=deg  RotationMatrix=[1 0 0;0 1 0;0 0 1]  Quaternion=[1 0 0 0]  TranslationMethod=StandardAxis  TranslationCartesianOffset=[0 0 0]  TranslationCartesianOffsetUnits=m  TranslationStandardAxis=+Z  TranslationStandardOffset=T  TranslationStandardOffsetUnits=cm  TranslationROffset=0  TranslationROffsetUnits=m  TranslationThetaOffset=0  TranslationThetaOffsetUnits=deg  TranslationZOffset=0  TranslationZOffsetUnits=m
  Connection Port : PMIOPort  Side=Left
  Connection Port1 : PMIOPort  Port=2  Side=Right
  connections:
  Connection Port/RConn1 -- Rigid Transform2/LConn1
  Connection Port1/RConn1 -- Rigid Transform/RConn1 -- Cylindrical Solid/RConn1
  Rigid Transform/LConn1 -- Extruded Solid1/LConn1 -- Rigid Transform2/RConn1 -- Extruded Solid/RConn1

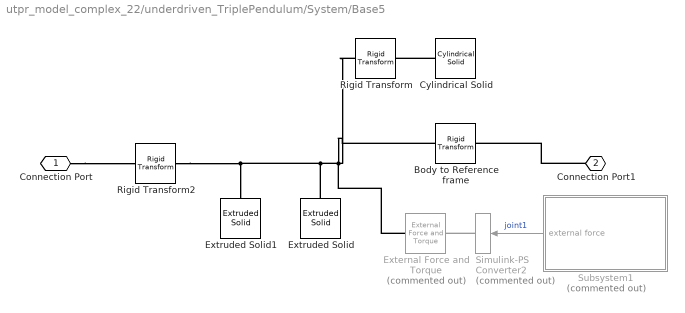
== system utpr_model_complex_22/underdriven_TriplePendulum/System/Base5 ==
  Body to Reference frame : sm_lib/Frames and Transforms/Rigid Transform  RotationMethod=None  FollAlignAxisA=+X  BaseAlignAxisA=+Y  FollAlignAxisB=+Y  BaseAlignAxisB=+Z  RotationStandardAxis=-Z  RotationAngle=90  RotationAngleUnits=deg  RotationArbitraryAxis=[0 0 1]  RotationSequenceAxes=FollowerAxes  RotationSequence=XYX  RotationSequenceAngles=[0 0 0]  RotationSequenceAnglesUnits=deg  RotationMatrix=[1 0 0; 0 1 0; 0 0 1]  Quaternion=[1 0 0 0]  TranslationMethod=StandardAxis  TranslationCartesianOffset=[0 0 0]  TranslationCartesianOffsetUnits=m  TranslationStandardAxis=+X  TranslationStandardOffset=L3  TranslationStandardOffsetUnits=m  TranslationROffset=0  TranslationROffsetUnits=m  TranslationThetaOffset=0  TranslationThetaOffsetUnits=deg  TranslationZOffset=0  TranslationZOffsetUnits=m
  Cylindrical Solid : sm_lib/Body Elements/Cylindrical Solid  CylinderRadius=0.03  CylinderRadiusUnits=m  CylinderLength=0.01  CylinderLengthUnits=m  ExportEntireGeometry=off  InertiaType=Custom  BasedOnType=Density  Density=1000  DensityUnits=kg/m^3  Mass=1e-20  MassUnits=kg  CenterOfMass=[0 0 0]  CenterOfMassUnits=m  MomentsOfInertia=[0 0 0]  MomentsOfInertiaUnits=kg*m^2  ProductsOfInertia=[0 0 0]  ProductsOfInertiaUnits=kg*m^2  GraphicType=FromGeometry  MarkerShape=Sphere  MarkerSize=10  GraphicVisPropType=SimpleVisualProperties  GraphicDiffuseColor=[0.0 0.6 0.0]  GraphicOpacity=1  GraphicSpecularColor=[0.5 0.5 0.5 1.0]  GraphicAmbientColor=[0.15 0.15 0.15 1.0]  GraphicEmissiveColor=[0.0 0.0 0.0 1.0]  GraphicShininess=75  DoExposeReferenceFrame=on  SerializedFrames=<Frames/>
  External Force and Torque : sm_lib/Forces and Torques/External Force and Torque  Commented=on  EnableForceX=on  EnableForceY=off  EnableForceZ=off  EnableForce=off  ForceResolutionFrame=World  EnableTorqueX=off  EnableTorqueY=off  EnableTorqueZ=off  EnableTorque=off  TorqueResolutionFrame=AttachedFrame
  Extruded Solid : sm_lib/Body Elements/Extruded Solid  ExtrusionType=General  PolygonNumSides=6  PolygonOuterRadius=R  PolygonOuterRadiusUnits=cm  ExportEntireGeometry=off  ExtrusionCrossSection=link3_section  ExtrusionCrossSectionUnits=m  ExportConvexHullGeometry=off  ExtrusionLength=T  ExtrusionLengthUnits=cm  InertiaType=Custom  BasedOnType=Density  Density=1  DensityUnits=kg/m^3  Mass=link3_m  MassUnits=kg  CenterOfMass=link3_CM  CenterOfMassUnits=m  MomentsOfInertia=link3_MI  MomentsOfInertiaUnits=kg*m^2  ProductsOfInertia=[0 0 0]  ProductsOfInertiaUnits=kg*m^2  GraphicType=FromGeometry  MarkerShape=Sphere  MarkerSize=10  GraphicVisPropType=SimpleVisualProperties  GraphicDiffuseColor=link1_rgb  GraphicOpacity=1  GraphicSpecularColor=[0.5 0.5 0.5 1.0]  GraphicAmbientColor=[0.15 0.15 0.15 1.0]  GraphicEmissiveColor=[0.0 0.0 0.0 1.0]  GraphicShininess=75  DoExposeReferenceFrame=on  SerializedFrames=<Frames/>
  Extruded Solid1 : sm_lib/Body Elements/Extruded Solid  ExtrusionType=General  PolygonNumSides=6  PolygonOuterRadius=R  PolygonOuterRadiusUnits=cm  ExportEntireGeometry=off  ExtrusionCrossSection=left_end_x_section  ExtrusionCrossSectionUnits=m  ExportConvexHullGeometry=off  ExtrusionLength=T  ExtrusionLengthUnits=cm  InertiaType=PointMass  BasedOnType=Density  Density=1  DensityUnits=kg/m^3  Mass=1e-20  MassUnits=g  CenterOfMass=[0 0 0]  CenterOfMassUnits=m  MomentsOfInertia=[1 1 1]  MomentsOfInertiaUnits=kg*m^2  ProductsOfInertia=[0 0 0]  ProductsOfInertiaUnits=kg*m^2  GraphicType=FromGeometry  MarkerShape=Sphere  MarkerSize=10  GraphicVisPropType=SimpleVisualProperties  GraphicDiffuseColor=link1_rgb  GraphicOpacity=1  GraphicSpecularColor=[0.5 0.5 0.5 1.0]  GraphicAmbientColor=[0.15 0.15 0.15 1.0]  GraphicEmissiveColor=[0.0 0.0 0.0 1.0]  GraphicShininess=75  DoExposeReferenceFrame=off  SerializedFrames=<Frames><Frame><Id>Frame1</Id><Value><Name>F1</Name><Origin><Source>ReferenceFrame</Source><FeatureName></FeatureName></Origin><PrimaryAxis><DefinedDirection>+Z</DefinedDirection><Source>ReferenceFrame</Source><SourceDirection>+Z</SourceDirection><FeatureName></FeatureName></PrimaryAxis><SecondaryAxis><DefinedDirection>+X</DefinedDirection><Source>ReferenceFrame</Source><SourceDirection>-X</SourceDirection><FeatureName></FeatureName></SecondaryAxis></Value></Frame></Frames>
  Rigid Transform : sm_lib/Frames and Transforms/Rigid Transform  RotationMethod=None  FollAlignAxisA=+X  BaseAlignAxisA=+Y  FollAlignAxisB=+Y  BaseAlignAxisB=+Z  RotationStandardAxis=+Z  RotationAngle=0  RotationAngleUnits=deg  RotationArbitraryAxis=[0 0 1]  RotationSequenceAxes=FollowerAxes  RotationSequence=XYX  RotationSequenceAngles=[0 0 0]  RotationSequenceAnglesUnits=deg  RotationMatrix=[1 0 0;0 1 0;0 0 1]  Quaternion=[1 0 0 0]  TranslationMethod=StandardAxis  TranslationCartesianOffset=[0 0 0]  TranslationCartesianOffsetUnits=m  TranslationStandardAxis=+X  TranslationStandardOffset=L3  TranslationStandardOffsetUnits=m  TranslationROffset=0  TranslationROffsetUnits=m  TranslationThetaOffset=0  TranslationThetaOffsetUnits=deg  TranslationZOffset=0  TranslationZOffsetUnits=m
  Rigid Transform2 : sm_lib/Frames and Transforms/Rigid Transform  RotationMethod=None  FollAlignAxisA=+X  BaseAlignAxisA=+X  FollAlignAxisB=-Y  BaseAlignAxisB=+Y  RotationStandardAxis=+Z  RotationAngle=90  RotationAngleUnits=deg  RotationArbitraryAxis=[0 0 1]  RotationSequenceAxes=FollowerAxes  RotationSequence=XYX  RotationSequenceAngles=[0 0 0]  RotationSequenceAnglesUnits=deg  RotationMatrix=[1 0 0;0 1 0;0 0 1]  Quaternion=[1 0 0 0]  TranslationMethod=StandardAxis  TranslationCartesianOffset=[0 0 0]  TranslationCartesianOffsetUnits=m  TranslationStandardAxis=+Z  TranslationStandardOffset=T  TranslationStandardOffsetUnits=cm  TranslationROffset=0  TranslationROffsetUnits=m  TranslationThetaOffset=0  TranslationThetaOffsetUnits=deg  TranslationZOffset=0  TranslationZOffsetUnits=m
  Simulink-PS Converter2 : nesl_utility/Simulink-PS Converter  Commented=on  PhysicalDomain=network_engine_domain  SubClassName=ps_input  LeftPortType=input  RightPortType=output  PseudoPeriodic=off  Frequencies=[]  NoiseDistribution=none  NoiseParameters=[]  Unit=1  AffineConversion=off  FilteringAndDerivatives=provide  SimscapeFilterOrder=2  InputFilterTimeConstant=0.001  UdotUserProvided=0
  Subsystem1 : Subsystem  Commented=on
  Connection Port : PMIOPort  Side=Left
  Connection Port1 : PMIOPort  Port=2  Side=Right
  wires:
  Subsystem1/1(external force) -> Simulink-PS Converter2/1  "joint1"
  connections:
  Connection Port/RConn1 -- Rigid Transform2/LConn1
  Connection Port1/RConn1 -- Body to Reference frame/RConn1
  Rigid Transform2/RConn1 -- External Force and Torque/RConn1 -- Rigid Transform/LConn1 -- Body to Reference frame/LConn1 -- Extruded Solid/RConn1 -- Extruded Solid1/LConn1
  Simulink-PS Converter2/RConn1 -- External Force and Torque/LConn1
  Cylindrical Solid/RConn1 -- Rigid Transform/RConn1

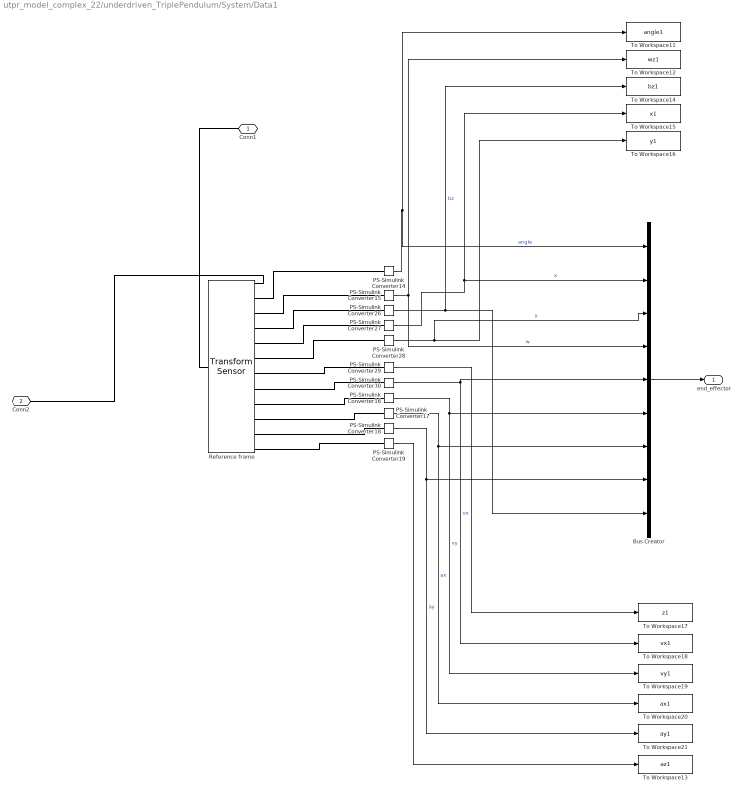
== system utpr_model_complex_22/underdriven_TriplePendulum/System/Data1 ==
  Bus Creator : BusCreator  Inputs=9
  PS-Simulink Converter{14..19,26..30} (11 alike) : nesl_utility/PS-Simulink Converter  PhysicalDomain=network_engine_domain  SubClassName=ps_output  LeftPortType=input  RightPortType=output  PseudoPeriodic=off  Frequencies=[]  VectorFormat=inherit  Unit=inherit  AffineConversion=off
  Reference frame : sm_lib/Frames and Transforms/Transform Sensor  MeasurementFrame=Base  RotationSequence=XYX  SenseAngle=on  SenseAxis=off  SenseQ=off  SenseR=off  SenseRotationSequence=off  SenseOmegaX=off  SenseOmegaY=off  SenseOmegaZ=on  SenseOmega=off  SenseQDot=off  SenseRDot=off  SenseRotationSequenceDot=off  SenseAlphaX=off  SenseAlphaY=off  SenseAlphaZ=on  SenseAlpha=off  SenseQDDot=off  SenseRDDot=off  SenseX=on  SenseY=on  SenseZ=on  SenseXYZ=off  SenseRad=off  SenseAzim=off  SenseDist=off  SenseInc=off  SenseXDot=on  SenseYDot=on  SenseZDot=off  SenseXYZDot=off  SenseRadDot=off  SenseAzimDot=off  SenseDistDot=off  SenseIncDot=off  SenseXDDot=on  SenseYDDot=on  SenseZDDot=on  SenseXYZDDot=off  SenseRadDDot=off  SenseAzimDDot=off  SenseDistDDot=off  SenseIncDDot=off
  To Workspace11 : ToWorkspace  VariableName=angle1  SaveFormat=Structure With Time  SampleTime=-1
  To Workspace12 : ToWorkspace  VariableName=wz1  SaveFormat=Structure With Time  SampleTime=-1
  To Workspace13 : ToWorkspace  VariableName=az1  SaveFormat=Structure With Time  SampleTime=-1
  To Workspace14 : ToWorkspace  VariableName=bz1  SaveFormat=Structure With Time  SampleTime=-1
  To Workspace15 : ToWorkspace  VariableName=x1  SaveFormat=Structure With Time  SampleTime=-1
  To Workspace16 : ToWorkspace  VariableName=y1  SaveFormat=Structure With Time  SampleTime=-1
  To Workspace17 : ToWorkspace  VariableName=z1  SaveFormat=Structure With Time  SampleTime=-1
  To Workspace18 : ToWorkspace  VariableName=vx1  SaveFormat=Structure With Time  SampleTime=-1
  To Workspace19 : ToWorkspace  VariableName=vy1  SaveFormat=Structure With Time  SampleTime=-1
  To Workspace20 : ToWorkspace  VariableName=ax1  SaveFormat=Structure With Time  SampleTime=-1
  To Workspace21 : ToWorkspace  VariableName=ay1  SaveFormat=Structure With Time  SampleTime=-1
  Conn1 : PMIOPort  Side=Left
  Conn2 : PMIOPort  Port=2  Side=Right
  end_effector : Outport
  wires:
  PS-Simulink Converter26/1 -> Bus Creator/9, To Workspace14/1  "bz"
  PS-Simulink Converter17/1 -> Bus Creator/7, To Workspace20/1  "ax"
  PS-Simulink Converter18/1 -> Bus Creator/8, To Workspace21/1  "ay"
  PS-Simulink Converter15/1 -> To Workspace12/1, Bus Creator/4  "w"
  PS-Simulink Converter27/1 -> Bus Creator/2, To Workspace15/1  "x"
  PS-Simulink Converter29/1 -> To Workspace17/1
  PS-Simulink Converter19/1 -> To Workspace13/1
  PS-Simulink Converter14/1 -> Bus Creator/1, To Workspace11/1  "angle"
  PS-Simulink Converter16/1 -> To Workspace19/1, Bus Creator/6  "vy"
  PS-Simulink Converter28/1 -> To Workspace16/1, Bus Creator/3  "y"
  PS-Simulink Converter30/1 -> To Workspace18/1, Bus Creator/5  "vx"
  Bus Creator/1 -> end_effector/1
  connections:
  Reference frame/RConn3 -- PS-Simulink Converter15/LConn1
  Reference frame/RConn7 -- PS-Simulink Converter29/LConn1
  Reference frame/RConn6 -- PS-Simulink Converter28/LConn1
  Reference frame/RConn8 -- PS-Simulink Converter30/LConn1
  Reference frame/RConn9 -- PS-Simulink Converter16/LConn1
  Reference frame/RConn11 -- PS-Simulink Converter18/LConn1
  Reference frame/RConn4 -- PS-Simulink Converter26/LConn1
  PS-Simulink Converter14/LConn1 -- Reference frame/RConn2
  Reference frame/RConn10 -- PS-Simulink Converter17/LConn1
  Reference frame/RConn5 -- PS-Simulink Converter27/LConn1
  Reference frame/RConn1 -- Conn2/RConn1
  Conn1/RConn1 -- Reference frame/LConn1
  Reference frame/RConn12 -- PS-Simulink Converter19/LConn1

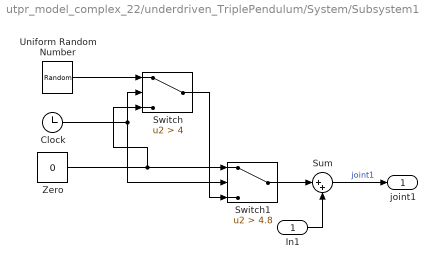
== system utpr_model_complex_22/underdriven_TriplePendulum/System/Subsystem1 ==
  In1 : Inport
  Clock : Clock
  Sum : Sum  Inputs=|++
  Switch : Switch  Criteria=u2 > Threshold  Threshold=4  SaturateOnIntegerOverflow=off  InputSameDT=off
  Switch1 : Switch  Criteria=u2 > Threshold  Threshold=4.8  SaturateOnIntegerOverflow=off  InputSameDT=off
  Uniform Random Number : UniformRandomNumber  Minimum=-0.003  Maximum=0.003  SampleTime=0.01
  Zero : Constant  Value=0  OutDataTypeStr=Inherit: Inherit via back propagation
  joint1 : Outport
  wires:
  Sum/1 -> joint1/1  "joint1"
  Switch/1 -> Switch1/3
  Zero/1 -> Switch/3, Switch1/1
  Clock/1 -> Switch1/2, Switch/2
  In1/1 -> Sum/2
  Switch1/1 -> Sum/1
  Uniform Random Number/1 -> Switch/1

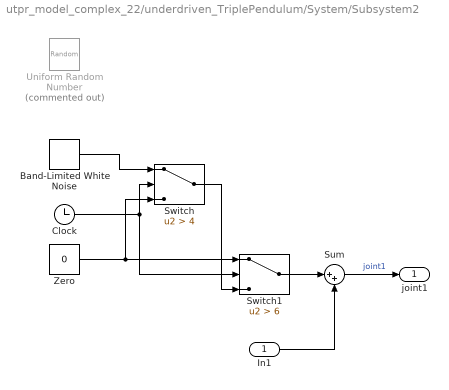
== system utpr_model_complex_22/underdriven_TriplePendulum/System/Subsystem2 ==
  In1 : Inport
  Band-Limited White Noise : simulink/Sources/Band-Limited White Noise  Cov=[0.01*0.01*0.01]  Ts=0.01  seed=[23341]
  Clock : Clock
  Sum : Sum  Inputs=|++
  Switch : Switch  Criteria=u2 > Threshold  Threshold=4  SaturateOnIntegerOverflow=off  InputSameDT=off
  Switch1 : Switch  Criteria=u2 > Threshold  Threshold=6  SaturateOnIntegerOverflow=off  InputSameDT=off
  Uniform Random Number : UniformRandomNumber  Commented=on  Minimum=-0.02  Maximum=0.02  SampleTime=0.01
  Zero : Constant  Value=0  OutDataTypeStr=Inherit: Inherit via back propagation
  joint1 : Outport
  wires:
  Sum/1 -> joint1/1  "joint1"
  Switch/1 -> Switch1/3
  Zero/1 -> Switch1/1, Switch/3
  Clock/1 -> Switch1/2, Switch/2
  In1/1 -> Sum/2
  Switch1/1 -> Sum/1
  Band-Limited White Noise/1 -> Switch/1

== system utpr_model_complex_22/underdriven_TriplePendulum/System/Base5/Subsystem1 ==
  Clock : Clock
  Constant : Constant  Value=3
  Switch : Switch  Criteria=u2 > Threshold  Threshold=5  SaturateOnIntegerOverflow=off  InputSameDT=off
  Switch1 : Switch  Criteria=u2 > Threshold  Threshold=5.1  SaturateOnIntegerOverflow=off  InputSameDT=off
  Zero : Constant  Value=0  OutDataTypeStr=Inherit: Inherit via back propagation
  external force : Outport
  wires:
  Switch/1 -> Switch1/3
  Zero/1 -> Switch/3, Switch1/1
  Clock/1 -> Switch1/2, Switch/2
  Switch1/1 -> external force/1
  Constant/1 -> Switch/1
